simulink model "controllo_test"  (R2020a)
settings: Solver=VariableStepAuto  StartTime=0.0  StopTime=100  RelTol=1e-3
values from neighbouring files (symbols this model uses):
  a = 0.35    [data.m]    (also in geodetic2nedS.m = 6378137)
  a1 = rho * D^4 * alpha1    (= 0.000388302366464)    [data.m]
  a2 = -rho * D^3 * alpha2 * (1 - omega)    (= 0.0037030698432)    [data.m]
  AHRS_bias = [0 0 0]    [data.m]
  AHRS_sample_time = 1/50    (= 0.02)    [data.m]
  AHRS_var = ([1 1 2] * pi/180).^2    [data.m]
  alpha1 = 0.0113    [data.m]
  alpha2 = -0.0091    [data.m]
  c = son2(1)    [Sonar_id.m]    (also in data.m = 0.19)
  current = [seaCurrent; 0; 0; 0]    [data.m]
  D = 0.076    [data.m]
  dead_zone_limit = 31.5    [data.m]
  DVL_sample_t = 1/12    (= 0.0833333333333)    [data.m]
  DVL_var1 = 0.005^2    (= 2.5e-05)    [data.m]
  DVL_var2 = 0.015^2    (= 0.000225)    [data.m]
  DVL_var3 = 0.023^2    (= 0.000529)    [data.m]
  gps_sample_t = 1    [data.m]
  H = eye(3)    [data.m]    (also in navigation_data.m)
  IMU_sample_time = 1/100    (= 0.01)    [data.m]
  initial = []    [data.m]
  INSP = unicode2native(inspectionDirection)    [data.m]
  Ki_bodypos1 = 0    [parametri_PID.m]
  Ki_bodypos2 = 0    [parametri_PID.m]
  Ki_bodypos3 = 0    [parametri_PID.m]
  Ki_bodypos4 = 0    [parametri_PID.m]
  Ki_bodypos5 = 0    [parametri_PID.m]
  Ki_depth1 = 0    [parametri_PID.m]
  Ki_depth2 = 0    [parametri_PID.m]
  Ki_depth3 = 0    [parametri_PID.m]
  Ki_depth4 = 0    [parametri_PID.m]
  Ki_depth5 = 0    [parametri_PID.m]
  Ki_latvel1 = 0    [parametri_PID.m]
  Ki_latvel2 = 0    [parametri_PID.m]
  Ki_latvel3 = 0    [parametri_PID.m]
  Ki_latvel4 = 0    [parametri_PID.m]
  Ki_latvel5 = 0    [parametri_PID.m]
  Ki_P1 = 0    [parametri_PID.m]
  Ki_P2 = 0    [parametri_PID.m]
  Ki_P3 = 0    [parametri_PID.m]
  Ki_P4 = 0    [parametri_PID.m]
  Ki_P5 = 0    [parametri_PID.m]
  Ki_R1 = 0    [parametri_PID.m]
  Ki_R2 = 0    [parametri_PID.m]
  Ki_R3 = 0    [parametri_PID.m]
  Ki_R4 = 0    [parametri_PID.m]
  Ki_R5 = 0    [parametri_PID.m]
  Ki_rel_or1 = 0    [parametri_PID.m]
  Ki_rel_or2 = 0    [parametri_PID.m]
  Ki_rel_or3 = 0    [parametri_PID.m]
  Ki_rel_or4 = 0    [parametri_PID.m]
  Ki_rel_or5 = 0    [parametri_PID.m]
  Ki_reldist1 = 0    [parametri_PID.m]
  Ki_reldist2 = 0    [parametri_PID.m]
  Ki_reldist3 = 0    [parametri_PID.m]
  Ki_reldist4 = 0    [parametri_PID.m]
  Ki_reldist5 = 0    [parametri_PID.m]
  Ki_surge1 = 0    [parametri_PID.m]
  Ki_surge2 = 0    [parametri_PID.m]
  Ki_surge3 = 0    [parametri_PID.m]
  Ki_surge4 = 0    [parametri_PID.m]
  Ki_surge5 = 0    [parametri_PID.m]
  Ki_yaw1 = 0    [parametri_PID.m]
  Ki_yaw2 = 0    [parametri_PID.m]
  Ki_yaw3 = 0    [parametri_PID.m]
  Ki_yaw4 = 0    [parametri_PID.m]
  Ki_yaw5 = 0    [parametri_PID.m]
  Kp_bodypos1 = 0    [parametri_PID.m]
  Kp_bodypos2 = 2    [parametri_PID.m]
  Kp_bodypos3 = 2    [parametri_PID.m]
  Kp_bodypos4 = 2    [parametri_PID.m]
  Kp_bodypos5 = 2    [parametri_PID.m]
  Kp_depth1 = 0    [parametri_PID.m]
  Kp_depth2 = 2    [parametri_PID.m]
  Kp_depth3 = 2    [parametri_PID.m]
  Kp_depth4 = 2    [parametri_PID.m]
  Kp_depth5 = 2    [parametri_PID.m]
  Kp_latvel1 = 0    [parametri_PID.m]
  Kp_latvel2 = 2    [parametri_PID.m]
  Kp_latvel3 = 2    [parametri_PID.m]
  Kp_latvel4 = 2    [parametri_PID.m]
  Kp_latvel5 = 2    [parametri_PID.m]
  Kp_P1 = 0    [parametri_PID.m]
  Kp_P2 = 2    [parametri_PID.m]
  Kp_P3 = 2    [parametri_PID.m]
  Kp_P4 = 2    [parametri_PID.m]
  Kp_P5 = 2    [parametri_PID.m]
  Kp_R1 = 0    [parametri_PID.m]
  Kp_R2 = 2    [parametri_PID.m]
  Kp_R3 = 2    [parametri_PID.m]
  Kp_R4 = 2    [parametri_PID.m]
  Kp_R5 = 2    [parametri_PID.m]
  Kp_rel_or1 = 0    [parametri_PID.m]
  Kp_rel_or2 = 2    [parametri_PID.m]
  Kp_rel_or3 = 2    [parametri_PID.m]
  Kp_rel_or4 = 2    [parametri_PID.m]
  Kp_rel_or5 = 2    [parametri_PID.m]
  Kp_reldist1 = 0    [parametri_PID.m]
  Kp_reldist2 = 2    [parametri_PID.m]
  Kp_reldist3 = 2    [parametri_PID.m]
  Kp_reldist4 = 2    [parametri_PID.m]
  Kp_reldist5 = 2    [parametri_PID.m]
  Kp_surge1 = 0    [parametri_PID.m]
  Kp_surge2 = 2    [parametri_PID.m]
  Kp_surge3 = 2    [parametri_PID.m]
  Kp_surge4 = 2    [parametri_PID.m]
  Kp_surge5 = 2    [parametri_PID.m]
  Kp_yaw1 = 0.6*6    (= 3.6)    [parametri_PID.m]
  Kp_yaw2 = 2    [parametri_PID.m]
  Kp_yaw3 = 2    [parametri_PID.m]
  Kp_yaw4 = 2    [parametri_PID.m]
  Kp_yaw5 = 2    [parametri_PID.m]
  M = M_rb + M_a    [Masse.m]
  M_inv = inv(M)    [Masse.m]
  n_max = 340    [data.m]
  num_cycle = 5    [data.m]    (also in navigation_data.m)
  omega = 0.1    [data.m]
  ps_sample_t = 0.02    [data.m]
  ps_var = (5000/3)^2    (= 2777777.77778)    [data.m]
  pylonCenter = [ 43.723046 ... (first row only)    [missionB.m]
  pylonRadius = 10    [missionB.m]
  ... (+3 more)
undefined symbols (not defined in the file or in its folder): arrival_point, DiscIntNeverNeededParam, Kd_bodypos2, Kd_bodyposy2, Kd_dist_mis2, Kd_surge2, Kd_yaw1, Ki_bodyposy2, Ki_dist_mis2, Kp_dist_mis2, s_data
libraries: simulink x8
(part 3 of 4)

== system controllo_test/Controller/ROTAZIONE IN SUPERFICIE/PID_YAW ==
  yaw_err : Inport
  "EN8 " : Inport  Port=2
  rel_or_err : Inport  Port=3
  EN7 : Inport  Port=4
  Constant : Constant  Value=0
  Constant1 : Constant  Value=0
  Discrete-Time Integrator : DiscreteIntegrator  ExternalReset=falling  SampleTime=0.1  ICPrevOutput=DiscIntNeverNeededParam  ICPrevScaledInput=DiscIntNeverNeededParam
  Discrete-Time Integrator1 : DiscreteIntegrator  ExternalReset=falling  SampleTime=0.1  ICPrevOutput=DiscIntNeverNeededParam  ICPrevScaledInput=DiscIntNeverNeededParam
  Gain : Gain  Gain=Kp_yaw3
  Gain1 : Gain  Gain=Kp_rel_or3
  Gain2 : Gain  Gain=Ki_yaw3
  Gain3 : Gain  Gain=Ki_rel_or3
  Sum : Sum  Inputs=++|
  Sum1 : Sum  Inputs=++|
  Switch : Switch  Criteria=u2 > Threshold  Threshold=0.5
  Switch1 : Switch  Criteria=u2 > Threshold  Threshold=0.5
  tau_yaw : Outport
  tau_rel_or : Outport  Port=2
  wires:
  Sum/1 -> tau_yaw/1
  Discrete-Time Integrator/1 -> Sum/2
  Switch/1 -> Gain/1, Gain2/1
  yaw_err/1 -> Switch/1
  Gain/1 -> Sum/1
  "EN8 "/1 -> [EN8], Switch/2
  Constant/1 -> Switch/3
  Gain2/1 -> Discrete-Time Integrator/1
  [EN8] -> Discrete-Time Integrator/2
  Discrete-Time Integrator1/1 -> Sum1/2
  [EN7] -> Discrete-Time Integrator1/2
  rel_or_err/1 -> Switch1/1
  EN7/1 -> [EN7], Switch1/2
  Switch1/1 -> Gain1/1, Gain3/1
  Sum1/1 -> tau_rel_or/1
  Constant1/1 -> Switch1/3
  Gain3/1 -> Discrete-Time Integrator1/1
  Gain1/1 -> Sum1/1

== system controllo_test/Env. & Sensor Model/AHRS SENSOR/Accelerometer ==
  note: Noise Density: < 0.14 mg/√Hz
  In1 : Inport
  Band-Limited White Noise : simulink/Sources/Band-Limited White Noise  Cov=acc_noise  Ts=IMU_sample_time  seed=[23341]
  Bias : Bias  Bias=0.0
  Sum : Sum  Inputs=|++
  lin_acc : Outport
  wires:
  Band-Limited White Noise/1 -> Sum/2
  Sum/1 -> lin_acc/1
  Bias/1 -> Sum/1
  In1/1 -> Bias/1

== system controllo_test/Env. & Sensor Model/AHRS SENSOR/Gyroscope ==
  note: Noise Density: 0.0035 °/s √Hz
  In1 : Inport
  Band-Limited White Noise : simulink/Sources/Band-Limited White Noise  Cov=gyro_noise  Ts=IMU_sample_time  seed=[341]
  Bias : Bias  Bias=0.0
  Sum : Sum  Inputs=|++
  ang_vel : Outport
  wires:
  Band-Limited White Noise/1 -> Sum/2
  Sum/1 -> ang_vel/1
  Bias/1 -> Sum/1
  In1/1 -> Bias/1

== system controllo_test/Env. & Sensor Model/AHRS SENSOR/Magnetometer ==
  note: Noise Density: 140 μGauss/√Hz
  In1 : Inport
  Band-Limited White Noise : simulink/Sources/Band-Limited White Noise  Cov=magn_noise  Ts=IMU_sample_time  seed=[31]
  Bias : Bias  Bias=0.0
  Sum : Sum  Inputs=|++
  m : Outport
  wires:
  Band-Limited White Noise/1 -> Sum/2
  Sum/1 -> m/1
  Bias/1 -> Sum/1
  In1/1 -> Bias/1

== system controllo_test/Env. & Sensor Model/DVL SENSOR/Subsystem ==
  In1 : Inport
  Abs : Abs
  Random Number : RandomNumber  Variance=DVL_var3  Seed=1  SampleTime=DVL_sample_t
  Random Number1 : RandomNumber  Variance=DVL_var2  Seed=2  SampleTime=DVL_sample_t
  Random Number2 : RandomNumber  Variance=DVL_var1  Seed=3  SampleTime=DVL_sample_t
  Switch2 : Switch  Criteria=u2 > Threshold  Threshold=2
  Switch3 : Switch  Criteria=u2 > Threshold  Threshold=4
  Out1 : Outport
  wires:
  Switch3/1 -> Switch2/1
  Random Number1/1 -> Switch3/3
  Random Number2/1 -> Switch2/3
  In1/1 -> Abs/1
  Switch2/1 -> Out1/1
  Random Number/1 -> Switch3/1
  Abs/1 -> Switch3/2, Switch2/2

== system controllo_test/Env. & Sensor Model/DVL SENSOR/Subsystem1 ==
  In1 : Inport
  Abs : Abs
  Random Number : RandomNumber  Variance=DVL_var3  Seed=4  SampleTime=DVL_sample_t
  Random Number1 : RandomNumber  Variance=DVL_var2  Seed=5  SampleTime=DVL_sample_t
  Random Number2 : RandomNumber  Variance=DVL_var1  Seed=2  SampleTime=DVL_sample_t
  Switch2 : Switch  Criteria=u2 > Threshold  Threshold=2
  Switch3 : Switch  Criteria=u2 > Threshold  Threshold=4
  Out1 : Outport
  wires:
  Switch3/1 -> Switch2/1
  Random Number1/1 -> Switch3/3
  Random Number2/1 -> Switch2/3
  In1/1 -> Abs/1
  Switch2/1 -> Out1/1
  Random Number/1 -> Switch3/1
  Abs/1 -> Switch3/2, Switch2/2

== system controllo_test/Env. & Sensor Model/DVL SENSOR/Subsystem2 ==
  In1 : Inport
  Abs : Abs
  Random Number : RandomNumber  Variance=DVL_var3  Seed=7  SampleTime=DVL_sample_t
  Random Number1 : RandomNumber  Variance=DVL_var2  Seed=2  SampleTime=DVL_sample_t
  Random Number2 : RandomNumber  Variance=DVL_var1  Seed=1  SampleTime=DVL_sample_t
  Switch2 : Switch  Criteria=u2 > Threshold  Threshold=2
  Switch3 : Switch  Criteria=u2 > Threshold  Threshold=4
  Out1 : Outport
  wires:
  Switch3/1 -> Switch2/1
  Random Number1/1 -> Switch3/3
  Random Number2/1 -> Switch2/3
  In1/1 -> Abs/1
  Switch2/1 -> Out1/1
  Random Number/1 -> Switch3/1
  Abs/1 -> Switch3/2, Switch2/2

== system controllo_test/Env. & Sensor Model/GPS SENSOR/Add noiose ==
  In1 : Inport
  In2 : Inport  Port=2
  Bus Creator : BusCreator  Inputs=2
  Random Number : RandomNumber  Variance=2  SampleTime=1
  Random Number1 : RandomNumber  Variance=2  Seed=332  SampleTime=1
  Sum2 : Sum  Inputs=|++
  Sum3 : Sum  Inputs=|++
  Out1 : Outport
  wires:
  In2/1 -> Sum3/1  "y in"
  Bus Creator/1 -> Out1/1  "out"
  In1/1 -> Sum2/1  "x in"
  Random Number/1 -> Sum2/2  "noise x"
  Random Number1/1 -> Sum3/2  "noise y"
  Sum2/1 -> Bus Creator/1  "x out"
  Sum3/1 -> Bus Creator/2  "y out"

== system controllo_test/Env. & Sensor Model/GPS SENSOR/Control state ==
  In1 : Inport
  AND : Logic  IconShape=distinctive  AllPortsSameDT=off  OutDataTypeStr=boolean
  Data Type Conversion : DataTypeConversion  OutDataTypeStr=double
  ENABLE GPS : Constant
  Zero-Order Hold : ZeroOrderHold  SampleTime=gps_sample_t
  Flag enable gps : Outport
  wires:
  ENABLE GPS/1 -> AND/2
  In1/1 -> AND/1
  AND/1 -> Data Type Conversion/1
  Data Type Conversion/1 -> Zero-Order Hold/1
  Zero-Order Hold/1 -> Flag enable gps/1

== system controllo_test/Env. & Sensor Model/Sonar sensor/Noises ==
  Mux : Mux  Inputs=s_data.num
  Random Number : RandomNumber  Mean=s_data.bias  Variance=s_data.noise^2  Seed=1  SampleTime=s_data.smpl  VectorParams1D=off
  Random Number1 : RandomNumber  Mean=s_data.bias  Variance=s_data.noise^2  Seed=2  SampleTime=s_data.smpl  VectorParams1D=off
  Random Number2 : RandomNumber  Mean=s_data.bias  Variance=s_data.noise^2  Seed=3  SampleTime=s_data.smpl  VectorParams1D=off
  Random Number3 : RandomNumber  Mean=s_data.bias  Variance=s_data.noise^2  Seed=4  SampleTime=s_data.smpl  VectorParams1D=off
  Random Number4 : RandomNumber  Mean=s_data.bias  Variance=s_data.noise^2  Seed=5  SampleTime=s_data.smpl  VectorParams1D=off
  Noises : Outport  SampleTime=s_data.smpl
  wires:
  Mux/1 -> Noises/1
  Random Number/1 -> Mux/1
  Random Number1/1 -> Mux/2
  Random Number2/1 -> Mux/3
  Random Number3/1 -> Mux/4
  Random Number4/1 -> Mux/5

== system controllo_test/Navigation1/Relative estimation/Sonar trigger ==
  In1 : Inport
  Demux : Demux  Outputs=[5 5]
  MATLAB Function : MATLAB Function  TreatAsAtomicUnit=on
  Scope2 : Scope
  Sum : Sum  Inputs=|+-
  Terminator : Terminator
  prev_sonar : Memory  InitialCondition=zeros(5,1)
  Out2 : Outport
  wires:
  Sum/1 -> MATLAB Function/2(sum)
  prev_sonar/1 -> Sum/2
  MATLAB Function/1(pulse) -> Out2/1, Scope2/1
  Demux/2 -> Terminator/1
  MATLAB Function/2(prev) -> prev_sonar/1
  In1/1 -> Demux/1
  Demux/1 -> MATLAB Function/1(sonar), Sum/1

== system controllo_test/Navigation1/Relative estimation/Subsystem ==
  Sonar : Inport
  Orientation : Inport  Port=2
  Trigger : TriggerPort  VariantControl=Variant  PortDimensions=1
  Demux : Demux  Outputs=[5 5]
  Display : Display
  Display1 : Display
  MATLAB Function9 : MATLAB Function  TreatAsAtomicUnit=on
  Terminator : Terminator
  Rel_distance : Outport  PortDimensions=1
  Rel_angle : Outport  Port=2  PortDimensions=1
  flag_sonar : Outport  Port=3  PortDimensions=1
  wires:
  Sonar/1 -> Demux/1, MATLAB Function9/1(sonar)
  MATLAB Function9/3(flag_sonar) -> Display/1, flag_sonar/1
  Orientation/1 -> MATLAB Function9/2(orientation)
  MATLAB Function9/2(alpha) -> Rel_angle/1
  MATLAB Function9/1(distance) -> Rel_distance/1
  Demux/1 -> Terminator/1
  Demux/2 -> Display1/1

== system controllo_test/Navigation1/z_EKF/EXTENDED KALMAN FILTER ==
  dT : Inport
  init : Inport  Port=2
  P0 : Inport  Port=3
  meas_pos : Inport  Port=4
  GPS_flag : Inport  Port=5
  meas_depth : Inport  Port=6
  orientation : Inport  Port=7
  dvl : Inport  Port=8
  ahrs_flag : Inport  Port=9
  Trigger : TriggerPort  VariantControl=Variant  PortDimensions=1
  "Correzione " : MATLAB Function  TreatAsAtomicUnit=on
  Demux : Demux  Outputs=[2 1]
  P : Memory  InitialCondition=zeros(3)  InheritSampleTime=on  StateName=P_pos
  Predizione : MATLAB Function  TreatAsAtomicUnit=on
  Scope : Scope
  hat_ : Memory  InitialCondition=zeros(3,1)  InheritSampleTime=on  StateName=P_pos
  previous_pos : Memory  InitialCondition=zeros(2,1)  InheritSampleTime=on  StateName=P_pos
  hat_pos : Outport
  hat_depth : Outport  Port=2
  wires:
  P/1 -> Predizione/1("P ")
  "Correzione "/2(P) -> P/1, Scope/1
  "Correzione "/1(prev_pos) -> previous_pos/1
  hat_/1 -> Predizione/2("hat ")
  "Correzione "/3(hat) -> Demux/1, hat_/1
  previous_pos/1 -> "Correzione "/1("prev_pos ")
  init/1 -> Predizione/7(init)
  orientation/1 -> Predizione/4(orientation)
  dT/1 -> Predizione/3(dT)
  dvl/1 -> Predizione/5(dvl)
  ahrs_flag/1 -> Predizione/6(ahrs_flag)
  P0/1 -> Predizione/8(P0)
  Predizione/1(P) -> "Correzione "/2("P ")
  Predizione/2(hat) -> "Correzione "/3("hat ")
  meas_pos/1 -> "Correzione "/4(meas_pos)
  GPS_flag/1 -> "Correzione "/5(GPS_flag)
  Demux/1 -> hat_pos/1
  Demux/2 -> hat_depth/1
  meas_depth/1 -> "Correzione "/6(meas_depth)

== system controllo_test/Navigation1/z_EKF/Trigger & Init ==
  meas_depth : Inport
  "meas_pos " : Inport  Port=2
  AND : Logic  IconShape=distinctive  AllPortsSameDT=off  OutDataTypeStr=boolean
  Depth trigger : Subsystem
  Initialization : Subsystem
  Scope{,1..3} (4 alike) : Scope
  pulse : Outport
  dT : Outport  Port=2
  init : Outport  Port=3
  P0 : Outport  Port=4
  wires:
  meas_depth/1 -> Depth trigger/1(Meas_depth), Initialization/1(Meas_depth)
  Depth trigger/2(Pulse) -> AND/1, Scope2/1
  "meas_pos "/1 -> Initialization/2(Meas_pos)
  Initialization/2(init) -> init/1, Scope3/1
  Initialization/3(P0) -> Scope/1, P0/1
  Depth trigger/1(dT) -> dT/1
  Initialization/1(pulse) -> AND/2, Scope1/1
  AND/1 -> pulse/1

== system controllo_test/Vehicle Model/Model Vehicle/Kinematic ==
  eta : Inport
  ni : Inport  Port=2
  Jac : MATLAB Function  TreatAsAtomicUnit=on
  Product : Product  Multiplication=Matrix(*)
  eta_dot : Outport  VectorParamsAs1DForOutWhenUnconnected=off
  wires:
  ni/1 -> Product/2
  Jac/1(J) -> Product/1
  eta/1 -> Jac/1(eta)
  Product/1 -> eta_dot/1

== system controllo_test/Vehicle Model/Thrusters/T ==
  des rot : Inport
  ni : Inport  Port=2
  Demux : Demux  Outputs=7
  Demux1 : Demux  Outputs=7
  MATLAB Function : MATLAB Function  TreatAsAtomicUnit=on
  Mux : Mux  Inputs=7
  Thruster 1 : Subsystem
  Thruster 2 : Subsystem
  Thruster 3 : Subsystem
  Thruster 4 : Subsystem
  Thruster 5 : Subsystem
  Thruster 6 : Subsystem
  Thruster 7 : Subsystem
  T : Outport  VectorParamsAs1DForOutWhenUnconnected=off
  wires:
  Demux/1 -> Thruster 1/1(n [rad/s])
  Demux/2 -> Thruster 2/1(n [rad/s])
  Demux/3 -> Thruster 3/1(n [rad/s])
  Demux/4 -> Thruster 4/1(n [rad/s])
  Demux/5 -> Thruster 5/1(n [rad/s])
  Demux/6 -> Thruster 6/1(n [rad/s])
  Demux/7 -> Thruster 7/1(n [rad/s])
  des rot/1 -> Demux/1
  Thruster 7/1(T i) -> Mux/7
  Thruster 6/1(T i) -> Mux/6
  Thruster 5/1(T i) -> Mux/5
  Thruster 4/1(T i) -> Mux/4
  Thruster 3/1(T i) -> Mux/3
  Thruster 2/1(T i) -> Mux/2
  Thruster 1/1(T i) -> Mux/1
  Mux/1 -> T/1
  MATLAB Function/1(v_th) -> Demux1/1
  Demux1/1 -> Thruster 1/2(V [m/s])
  Demux1/2 -> Thruster 2/2(V [m/s])
  Demux1/3 -> Thruster 3/2(V [m/s])
  Demux1/4 -> Thruster 4/2(V [m/s])
  Demux1/5 -> Thruster 5/2(V [m/s])
  Demux1/6 -> Thruster 6/2(V [m/s])
  Demux1/7 -> Thruster 7/2(V [m/s])
  ni/1 -> MATLAB Function/1(ni)

== system controllo_test/Navigation1/z_EKF/Trigger & Init/Depth trigger ==
  Meas_depth : Inport
  Demux : Demux  Outputs=2
  MATLAB Function : MATLAB Function  TreatAsAtomicUnit=on
  Sum : Sum  Inputs=|+-
  Terminator : Terminator
  count : Memory  InitialCondition=1
  prev_depth : Memory
  dT : Outport
  Pulse : Outport  Port=2
  wires:
  Sum/1 -> MATLAB Function/3(sum)
  prev_depth/1 -> Sum/2
  MATLAB Function/3(pulse) -> Pulse/1
  Demux/2 -> Terminator/1
  MATLAB Function/4(prev) -> prev_depth/1
  MATLAB Function/2(dT) -> dT/1
  Meas_depth/1 -> Demux/1
  count/1 -> MATLAB Function/1("count ")
  Demux/1 -> MATLAB Function/2(depth), Sum/1
  MATLAB Function/1(count) -> count/1

== system controllo_test/Navigation1/z_EKF/Trigger & Init/Initialization ==
  Meas_depth : Inport
  Meas_pos : Inport  Port=2
  Demux1 : Demux  Outputs=[2 1]
  Demux2 : Demux  Outputs=2
  MATLAB Function1 : MATLAB Function  TreatAsAtomicUnit=on
  Scope3 : Scope
  Sum1 : Sum  Inputs=|+-
  Terminator2 : Terminator
  init_counter : Memory
  prev_pos : Memory  InitialCondition=zeros(2,1)
  store_depth : Memory  InitialCondition=zeros(num_cycle,1)
  store_gps : Memory  InitialCondition=zeros(2,num_cycle)
  pulse : Outport
  init : Outport  Port=2
  P0 : Outport  Port=3
  wires:
  Demux1/1 -> MATLAB Function1/3(gps), Sum1/1
  MATLAB Function1/4(P0) -> P0/1
  MATLAB Function1/3(init) -> init/1
  MATLAB Function1/2(pulse) -> pulse/1, Scope3/1
  init_counter/1 -> MATLAB Function1/1("init_counter ")
  Sum1/1 -> MATLAB Function1/5(diff_)
  Demux2/1 -> MATLAB Function1/2(depth)
  MATLAB Function1/6(gps_store) -> store_gps/1
  MATLAB Function1/1(init_counter) -> init_counter/1
  Demux2/2 -> Terminator2/1
  MATLAB Function1/7(depth_store) -> store_depth/1
  store_gps/1 -> MATLAB Function1/6(store_gps)
  store_depth/1 -> MATLAB Function1/7(store_depth)
  Meas_depth/1 -> Demux2/1
  MATLAB Function1/5(prev) -> prev_pos/1
  prev_pos/1 -> Sum1/2
  Meas_pos/1 -> Demux1/1
  Demux1/2 -> MATLAB Function1/4(GPS_flag)

== system controllo_test/Vehicle Model/Thrusters/T/Thruster 1 ==
  note: n is the rotational speed of the thruster
      | V is the speed component of the water along the thruster axis
      |
      | n is saturated according to data
      | a dead zone is considered according to data
      | the thruster is characterised by 1st order dynamics (tau = 0.2s)
  n [rad/s] : Inport
  V [m/s] : Inport  Port=2
  Dead Zone : DeadZone  LowerValue=-dead_zone_limit  UpperValue=dead_zone_limit  SaturateOnIntegerOverflow=on
  MATLAB Function : MATLAB Function  TreatAsAtomicUnit=on
  Saturation : Saturate  UpperLimit=n_max  LowerLimit=-n_max
  Transfer Fcn : TransferFcn  Denominator=[0.2 1]
  T i : Outport
  wires:
  V [m/s]/1 -> MATLAB Function/2(V)
  Saturation/1 -> MATLAB Function/1(n)
  Transfer Fcn/1 -> Saturation/1
  Dead Zone/1 -> Transfer Fcn/1
  n [rad/s]/1 -> Dead Zone/1
  MATLAB Function/1(T) -> T i/1

== system controllo_test/Vehicle Model/Thrusters/T/Thruster 2 ==
  note: n is the rotational speed of the thruster
      | V is the speed component of the water along the thruster axis
      |
      | n is saturated according to data
      | a dead zone is considered according to data
      | the thruster is characterised by 1st order dynamics (tau = 0.2s)
  n [rad/s] : Inport
  V [m/s] : Inport  Port=2
  Dead Zone : DeadZone  LowerValue=-dead_zone_limit  UpperValue=dead_zone_limit  SaturateOnIntegerOverflow=on
  MATLAB Function : MATLAB Function  TreatAsAtomicUnit=on
  Saturation : Saturate  UpperLimit=n_max  LowerLimit=-n_max
  Transfer Fcn : TransferFcn  Denominator=[0.2 1]
  T i : Outport
  wires:
  V [m/s]/1 -> MATLAB Function/2(V)
  Saturation/1 -> MATLAB Function/1(n)
  Transfer Fcn/1 -> Saturation/1
  Dead Zone/1 -> Transfer Fcn/1
  n [rad/s]/1 -> Dead Zone/1
  MATLAB Function/1(T) -> T i/1

== system controllo_test/Vehicle Model/Thrusters/T/Thruster 3 ==
  note: n is the rotational speed of the thruster
      | V is the speed component of the water along the thruster axis
      |
      | n is saturated according to data
      | a dead zone is considered according to data
      | the thruster is characterised by 1st order dynamics (tau = 0.2s)
  n [rad/s] : Inport
  V [m/s] : Inport  Port=2
  Dead Zone : DeadZone  LowerValue=-dead_zone_limit  UpperValue=dead_zone_limit  SaturateOnIntegerOverflow=on
  MATLAB Function : MATLAB Function  TreatAsAtomicUnit=on
  Saturation : Saturate  UpperLimit=n_max  LowerLimit=-n_max
  Transfer Fcn : TransferFcn  Denominator=[0.2 1]
  T i : Outport
  wires:
  V [m/s]/1 -> MATLAB Function/2(V)
  Saturation/1 -> MATLAB Function/1(n)
  Transfer Fcn/1 -> Saturation/1
  Dead Zone/1 -> Transfer Fcn/1
  n [rad/s]/1 -> Dead Zone/1
  MATLAB Function/1(T) -> T i/1

== system controllo_test/Vehicle Model/Thrusters/T/Thruster 4 ==
  note: n is the rotational speed of the thruster
      | V is the speed component of the water along the thruster axis
      |
      | n is saturated according to data
      | a dead zone is considered according to data
      | the thruster is characterised by 1st order dynamics (tau = 0.2s)
  n [rad/s] : Inport
  V [m/s] : Inport  Port=2
  Dead Zone : DeadZone  LowerValue=-dead_zone_limit  UpperValue=dead_zone_limit  SaturateOnIntegerOverflow=on
  MATLAB Function : MATLAB Function  TreatAsAtomicUnit=on
  Saturation : Saturate  UpperLimit=n_max  LowerLimit=-n_max
  Transfer Fcn : TransferFcn  Denominator=[0.2 1]
  T i : Outport
  wires:
  V [m/s]/1 -> MATLAB Function/2(V)
  Saturation/1 -> MATLAB Function/1(n)
  Transfer Fcn/1 -> Saturation/1
  Dead Zone/1 -> Transfer Fcn/1
  n [rad/s]/1 -> Dead Zone/1
  MATLAB Function/1(T) -> T i/1

== system controllo_test/Vehicle Model/Thrusters/T/Thruster 5 ==
  note: n is the rotational speed of the thruster
      | V is the speed component of the water along the thruster axis
      |
      | n is saturated according to data
      | a dead zone is considered according to data
      | the thruster is characterised by 1st order dynamics (tau = 0.2s)
  n [rad/s] : Inport
  V [m/s] : Inport  Port=2
  Dead Zone : DeadZone  LowerValue=-dead_zone_limit  UpperValue=dead_zone_limit  SaturateOnIntegerOverflow=on
  MATLAB Function : MATLAB Function  TreatAsAtomicUnit=on
  Saturation : Saturate  UpperLimit=n_max  LowerLimit=-n_max
  Transfer Fcn : TransferFcn  Denominator=[0.2 1]
  T i : Outport
  wires:
  V [m/s]/1 -> MATLAB Function/2(V)
  Saturation/1 -> MATLAB Function/1(n)
  Transfer Fcn/1 -> Saturation/1
  Dead Zone/1 -> Transfer Fcn/1
  n [rad/s]/1 -> Dead Zone/1
  MATLAB Function/1(T) -> T i/1

== system controllo_test/Vehicle Model/Thrusters/T/Thruster 6 ==
  note: n is the rotational speed of the thruster
      | V is the speed component of the water along the thruster axis
      |
      | n is saturated according to data
      | a dead zone is considered according to data
      | the thruster is characterised by 1st order dynamics (tau = 0.2s)
  n [rad/s] : Inport
  V [m/s] : Inport  Port=2
  Dead Zone : DeadZone  LowerValue=-dead_zone_limit  UpperValue=dead_zone_limit  SaturateOnIntegerOverflow=on
  MATLAB Function : MATLAB Function  TreatAsAtomicUnit=on
  Saturation : Saturate  UpperLimit=n_max  LowerLimit=-n_max
  Transfer Fcn : TransferFcn  Denominator=[0.2 1]
  T i : Outport
  wires:
  V [m/s]/1 -> MATLAB Function/2(V)
  Saturation/1 -> MATLAB Function/1(n)
  Transfer Fcn/1 -> Saturation/1
  Dead Zone/1 -> Transfer Fcn/1
  n [rad/s]/1 -> Dead Zone/1
  MATLAB Function/1(T) -> T i/1

== system controllo_test/Vehicle Model/Thrusters/T/Thruster 7 ==
  note: n is the rotational speed of the thruster
      | V is the speed component of the water along the thruster axis
      |
      | n is saturated according to data
      | a dead zone is considered according to data
      | the thruster is characterised by 1st order dynamics (tau = 0.2s)
  n [rad/s] : Inport
  V [m/s] : Inport  Port=2
  Dead Zone : DeadZone  LowerValue=-dead_zone_limit  UpperValue=dead_zone_limit  SaturateOnIntegerOverflow=on
  MATLAB Function : MATLAB Function  TreatAsAtomicUnit=on
  Saturation : Saturate  UpperLimit=n_max  LowerLimit=-n_max
  Transfer Fcn : TransferFcn  Denominator=[0.2 1]
  T i : Outport
  wires:
  V [m/s]/1 -> MATLAB Function/2(V)
  Saturation/1 -> MATLAB Function/1(n)
  Transfer Fcn/1 -> Saturation/1
  Dead Zone/1 -> Transfer Fcn/1
  n [rad/s]/1 -> Dead Zone/1
  MATLAB Function/1(T) -> T i/1

== matlab function controllo_test/Vehicle Model/Thrusters/T/Thruster 3/MATLAB Function ==
  data: n input; T output; V input; D parameter; omega parameter; a1 parameter; a2 parameter; alpha1 parameter; alpha2 parameter
function T = thrusterModel(n, V, D, omega, a1, a2, alpha1, alpha2)

Va = (1-omega) * V;     % Advancement velocity at the propeller
J0 = Va/(n*D);          % Advancement Coefficient

if J0 > -alpha1/alpha2  % Out of linearity domain (right side)
    T = 0;              % A null generated thrust is assumed
    
elseif J0 < 0           % Out of linearity domain (left side)
    T = a1*abs(n)*n;    % Bollard thrust is assumed

else                    % Within the linearity domain
    T = a1*abs(n)*n - a2*abs(n)*V;
end

== matlab function controllo_test/Vehicle Model/Thrusters/T/Thruster 4/MATLAB Function ==
  data: n input; T output; V input; D parameter; omega parameter; a1 parameter; a2 parameter; alpha1 parameter; alpha2 parameter
function T = thrusterModel(n, V, D, omega, a1, a2, alpha1, alpha2)

Va = (1-omega) * V;     % Advancement velocity at the propeller
J0 = Va/(n*D);          % Advancement Coefficient

if J0 > -alpha1/alpha2  % Out of linearity domain (right side)
    T = 0;              % A null generated thrust is assumed
    
elseif J0 < 0           % Out of linearity domain (left side)
    T = a1*abs(n)*n;    % Bollard thrust is assumed

else                    % Within the linearity domain
    T = a1*abs(n)*n - a2*abs(n)*V;
end

== matlab function controllo_test/Vehicle Model/Thrusters/T/Thruster 5/MATLAB Function ==
  data: n input; T output; V input; D parameter; omega parameter; a1 parameter; a2 parameter; alpha1 parameter; alpha2 parameter
function T = thrusterModel(n, V, D, omega, a1, a2, alpha1, alpha2)

Va = (1-omega) * V;     % Advancement velocity at the propeller
J0 = Va/(n*D);          % Advancement Coefficient

if J0 > -alpha1/alpha2  % Out of linearity domain (right side)
    T = 0;              % A null generated thrust is assumed
    
elseif J0 < 0           % Out of linearity domain (left side)
    T = a1*abs(n)*n;    % Bollard thrust is assumed

else                    % Within the linearity domain
    T = a1*abs(n)*n - a2*abs(n)*V;
end

== matlab function controllo_test/Vehicle Model/Thrusters/T/Thruster 6/MATLAB Function ==
  data: n input; T output; V input; D parameter; omega parameter; a1 parameter; a2 parameter; alpha1 parameter; alpha2 parameter
function T = thrusterModel(n, V, D, omega, a1, a2, alpha1, alpha2)

Va = (1-omega) * V;     % Advancement velocity at the propeller
J0 = Va/(n*D);          % Advancement Coefficient

if J0 > -alpha1/alpha2  % Out of linearity domain (right side)
    T = 0;              % A null generated thrust is assumed
    
elseif J0 < 0           % Out of linearity domain (left side)
    T = a1*abs(n)*n;    % Bollard thrust is assumed

else                    % Within the linearity domain
    T = a1*abs(n)*n - a2*abs(n)*V;
end

== matlab function controllo_test/Vehicle Model/Thrusters/T/Thruster 7/MATLAB Function ==
  data: n input; T output; V input; D parameter; omega parameter; a1 parameter; a2 parameter; alpha1 parameter; alpha2 parameter
function T = thrusterModel(n, V, D, omega, a1, a2, alpha1, alpha2)

Va = (1-omega) * V;     % Advancement velocity at the propeller
J0 = Va/(n*D);          % Advancement Coefficient

if J0 > -alpha1/alpha2  % Out of linearity domain (right side)
    T = 0;              % A null generated thrust is assumed
    
elseif J0 < 0           % Out of linearity domain (left side)
    T = a1*abs(n)*n;    % Bollard thrust is assumed

else                    % Within the linearity domain
    T = a1*abs(n)*n - a2*abs(n)*V;
end

== matlab function controllo_test/Vehicle Model/Model Vehicle/MATLAB Function ==
  data: coord_pylon input; eta input; eta_ecef output
function eta_ecef = nedToEcef(coord_pylon, eta)

    coder.extrinsic('wgs84Ellipsoid');

    coder.extrinsic('ned2geodetic');
    
    eta_pos = eta(1:6);
    wgs84 = wgs84Ellipsoid('meter'); %TODO verificare che esprima le coordinate nello stesso modo dell'ECEF dato in missionB.m
    [eta_pos(1), eta_pos(2)] = ned2geodetic(eta(1), eta(2), eta(3), coord_pylon(1), coord_pylon(2), coord_pylon(3), wgs84,'degrees');
    
    eta_pos(3) = eta(3);
    eta_pos(4:6) = eta_pos(4:6);
    
    eta_ecef = eta_pos;
    
end

== matlab function controllo_test/Vehicle Model/MATLAB Function ==
  data: eta input; ni_c output; current input
function ni_c = current_ned2body(eta, current)
    eta2 = eta(4:6)*pi/180;     % eta2 espresso in radianti
    ni_c = Jac(eta2)'*current;
end

== matlab function controllo_test/Vehicle Model/Thrusters/T/MATLAB Function ==
  data: ni input; v_th output
function v_th = thrusters(ni)
p1 = [-0.35 -0.25 0]';
p2 = [-0.35 0.25 0]';
p3 = [-0.25 -0.35 0]';
p4 = [0.25 0.35 0]';
p5 = [-0.25 -0.25 -0.19]';
p6 = [-0.25 0.25 -0.19]';
p7 = [0.25 0 -0.19]';

t1 = [1 0 0]';
t2 = t1;
t3 = [0 1 0]';
t4 = -t3;
t5 = [0 0 1]';
t6 = t5;
t7 = t5;

v_lin = ni(1:3);
v_ang = ni(4:6);

vp1 = v_lin + cross(v_ang, p1);
vp2 = v_lin + cross(v_ang, p2);
vp3 = v_lin + cross(v_ang, p3);
vp4 = v_lin + cross(v_ang, p4);
vp5 = v_lin + cross(v_ang, p5);
vp6 = v_lin + cross(v_ang, p6);
vp7 = v_lin + cross(v_ang, p7);

v1 = vp1'*t1;
v2 = vp2'*t2;
v3 = vp3'*t3;
v4 = vp4'*t4;
v5 = vp5'*t5;
v6 = vp6'*t6;
v7 = vp7'*t7;

v_th = [ v1 v2 v3 v4 v5 v6 v7]';
end

== matlab function controllo_test/Navigation1/Geodetic to NED/MATLAB Function2 ==
  data: GPS_geodetic input; GPS_flag input; GPS_NED output; depth input; pylonCenter parameter
function GPS_NED = Geo2NED(GPS_geodetic, GPS_flag, depth, pylonCenter)

% Funzione che trasforma le coordinate dal sistema di riferimento geodetico
% ad un sistema NED con origine in corrispondenza del centro del pilone.

%% GPS non funzionante
if GPS_flag == 0            
    GPS_NED = [0;0;0];
    return
end

%% Variabili
phi = GPS_geodetic(1);                  % Coordinate geodetiche in radianti                     
lambda = GPS_geodetic(2);  
h = -depth;

phi_pyl = pylonCenter(1) * pi/180;      % Origine del sistema NED in coordinate geodetiche
lambda_pyl = pylonCenter(2) * pi/180;

%% Trasformazione coordinate
coder.extrinsic('wgs84Ellipsoid');
coder.extrinsic('geodetic2ned');
    
[x_gps2, y_gps2, z_gps2] = geodetic2ned(phi, lambda, -depth, phi_pyl, lambda_pyl, 0, wgs84Ellipsoid, 'radians');
eta_NED_GPS = [x_gps2; y_gps2];

GPS_NED = zeros(3,1);
GPS_NED(1) = eta_NED_GPS(1);            % Coordiante NED in radianti
GPS_NED(2) = eta_NED_GPS(2);
GPS_NED(3) = GPS_flag;

== matlab function controllo_test/Vehicle Model/Thrusters/saturation_tau ==
  data: tau input; tau_sat output; eta input
function tau_sat = sat_tau(tau, eta)
    tau_sat = [0;0;0;0;0;0];
    tau_sat = tau;

    if eta(3) < 0.1 %semiasse c
        tau_sat(3) = 0;
    end
    
end

== matlab function controllo_test/Navigation1/Geodetic to NED2/MATLAB Function2 ==
  data: GPS_geodetic input; GPS_flag input; GPS_NED output; depth input; pylonCenter parameter
function GPS_NED = Geo2NED(GPS_geodetic, GPS_flag, depth, pylonCenter)

% Funzione che trasforma le coordinate dal sistema di riferimento geodetico
% ad un sistema NED con origine in corrispondenza del centro del pilone.

%% GPS non funzionante
if GPS_flag == 0            
    GPS_NED = [0;0;0];
    return
end

%% Variabili
phi = GPS_geodetic(1);                  % Coordinate geodetiche in radianti                     
lambda = GPS_geodetic(2);  
h = -depth;

phi_pyl = pylonCenter(1) * pi/180;      % Origine del sistema NED in coordinate geodetiche
lambda_pyl = pylonCenter(2) * pi/180;

%% Trasformazione coordinate
coder.extrinsic('wgs84Ellipsoid');
coder.extrinsic('geodetic2ned');
    
[x_gps2, y_gps2, z_gps2] = geodetic2ned(phi, lambda, -depth, phi_pyl, lambda_pyl, 0, wgs84Ellipsoid, 'radians');
eta_NED_GPS = [x_gps2; y_gps2];

GPS_NED = zeros(3,1);
GPS_NED(1) = eta_NED_GPS(1);            % Coordiante NED in radianti
GPS_NED(2) = eta_NED_GPS(2);
GPS_NED(3) = GPS_flag;

== matlab function controllo_test/Navigation1/MATLAB Function1 ==
  data: ang_vel input; DVL input; nu_1 output; c parameter
function nu_1  = dvl2body(ang_vel, DVL, c)

% Funzione che si occupa di trasformare la velocità da sistema di
% riferimento associato al DVL al sistema BODY

% nu_dvl = R_b^dvl (nu_1 + S(nu_2)* P_dvl)
% nu_1 = R_b^dvl' * nu_dvl - S(nu_2) * P_dvl

nu_1    =   zeros(4,1);
nu_2    =   [ang_vel(1); ang_vel(2); ang_vel(3)];
vel_dvl =   [DVL(1); DVL(2); DVL(3)];
R_b_dvl =   eye(3);

S = [   0,          -nu_2(3),   nu_2(2); 
        nu_2(3),    0,          -nu_2(1); 
        -nu_2(2),   nu_2(1),    0       ];
    
p = [0;0;c];

nu_1(1:3) = R_b_dvl' * vel_dvl - S * p;
nu_1(4) = DVL(4); %Flag

== matlab function controllo_test/Navigation1/MATLAB Function2 ==
  data: Depth_ps input; Depth output; c parameter
function  Depth = ps2body(Depth_ps, c)
% Il profondimetro è posizionato nella parte inferiore dell'AUV, lungo
% l'asse z
Depth = zeros(2,1);
Depth(1) = Depth_ps(1) - c;     %profondità rispetto al centro di massa
Depth(2) = Depth_ps(2);         %flag

== matlab function controllo_test/Navigation1/AHRS_function ==
  data: eta2 output; lin_acc input; nu2 output; ang_vel input; orientation input
function [eta2, nu2]= AHRS_signals(lin_acc, ang_vel, orientation)
acc = lin_acc(1:3);
nu2 = ang_vel(1:3);
eta2 = orientation(1:3);

== matlab function controllo_test/Navigation1/DVL_function ==
  data: dvl input; velocity_est output; flag_DVL output
function [velocity_est, flag_DVL] = DVL_signals(dvl)
velocity_est = dvl(1:3);
flag_DVL = dvl(4);

== matlab function controllo_test/Navigation1/NED to Geodetic/MATLAB Function1 ==
  data: eta_NED input; eta_geodetic output; depth input; pylonCenter parameter
function eta_geodetic = NED2Geo(eta_NED, depth, pylonCenter)

% Funzione che trasforma le coordinate dal sistema NED con origine in
% corrispondenza del centro del pilone al sistema di riferimento geodetico

phi_pyl = pylonCenter(1) * pi/180;      % Origine del sistema NED in coordinate geodetiche 
lambda_pyl = pylonCenter(2) * pi/180;

%% Trasformazione
coder.extrinsic('wgs84Ellipsoid');
coder.extrinsic('ned2geodetic');

[lat, lon, h] = ned2geodetic(eta_NED(1), eta_NED(2), depth, phi_pyl, lambda_pyl, 0, wgs84Ellipsoid, 'radians');

eta_geodetic = [0; 0];
eta_geodetic = [lat; lon];              % Coordiante geodetiche in radianti

== matlab function controllo_test/Navigation1/Relative estimation/Sonar trigger/MATLAB Function ==
  data: sonar input; sum input; pulse output; prev output
function [pulse, prev] = fcn(sonar, sum)

% La funzione si occupa di monitorare la misura dei sonar,
% quando esse sono modificate manda un impulso al blocco di stima relativa

if nnz(isnan(sum)) > 0 || nnz(sum) == 0 
    pulse = 0;
else
    pulse = 1;
end

prev = sonar;

== matlab function controllo_test/Navigation1/Relative estimation/Subsystem/MATLAB Function9 ==
  data: sonar input; orientation input; distance output; alpha output; flag_sonar output; pylonRadius parameter; a parameter; s_data parameter
function [distance, alpha, flag_sonar] = relative_values(sonar, orientation, pylonRadius, a, s_data)

% Chiamando la funzione "fcn_sonar" si occupa di calcolate la distanza
% e l'angolo dell'AUV rispetto al pilone

distance = 0;
alpha = 0;
flag_sonar = 0;

coder.extrinsic('fcn_sonar');

[distance, alpha, flag_sonar] = fcn_sonar(sonar, orientation, pylonRadius, a, s_data);
end

== matlab function controllo_test/Navigation1/flag_function ==
  data: flag_depth input; flag_AHRS input; error_flag output; flag_DVL input; flag_sonar input
function error_flag = fcn(flag_depth, flag_AHRS, flag_DVL, flag_sonar)

% Funzione che rileva la presenza di errore in un sensore

flag_ahrs = flag_AHRS(1) & flag_AHRS(2) & flag_AHRS(3);
error_flag = ~(flag_depth & flag_ahrs & flag_DVL & flag_sonar); % Vale 1 se vi è un errore

== matlab function controllo_test/Navigation1/z_EKF/EXTENDED KALMAN FILTER/Correzione  ==
  data: prev_pos output; prev_pos input; P input; hat input; meas_pos input; GPS_flag input; meas_depth input; P output; hat output; R parameter; H parameter
function [prev_pos, P, hat] = EKF_pos(prev_pos, P, hat, meas_pos, GPS_flag, meas_depth, R, H)
%% EKF: Correction

% Il filtro corregge i valori di posizione x e y solo quando è disponibile una nuova misura del GPS
if nnz(round(10.^4*(meas_pos - prev_pos))/10.^4) ~= 0 && GPS_flag == 1       % Se il flag è 0 il GPS non funziona

    z_tilde = [ meas_pos(1) - hat(1);
                meas_pos(2) - hat(2);
                meas_depth - hat(3)];

else
        z_tilde = [ 0;
                    0;
                meas_depth - hat(3)];
end
            
    S = H * P * H' + R;

    K = P * H' * S^(-1);
    
    hat = hat + K * z_tilde;
    P = (eye(3) - K * H) * P;  

prev_pos = meas_pos;

== matlab function controllo_test/Navigation1/z_EKF/EXTENDED KALMAN FILTER/Predizione ==
  data: P input; hat input; dT input; P output; hat output; orientation input; dvl input; ahrs_flag input; init input; P0 input; Q parameter
function [P, hat]  = EKF_pos(P, hat, dT, orientation, dvl, ahrs_flag, init, P0, Q)

dvl_flag = dvl(4);

%% Inizializzazione stato e matrice P
if nnz(hat) == 0           
    hat= init;
    P = P0;
end

if (ahrs_flag && dvl_flag) == 1
    %% Calcolo variabili e matrici
    phi     =   orientation(1);             % roll
    theta   =   orientation(2);             % pitch
    psi_    =   orientation(3);             % yaw
    vel     =   [dvl(1); dvl(2); dvl(3)];  
    
    J       =   zeros(3,3);
    Lk      =   zeros(3,6);
    
    J = [ cos(psi_)*cos(theta), cos(psi_)*sin(phi)*sin(theta) - cos(phi)*sin(psi_), sin(phi)*sin(psi_) + cos(phi)*cos(psi_)*sin(theta);
       cos(theta)*sin(psi_), cos(phi)*cos(psi_) + sin(phi)*sin(psi_)*sin(theta), cos(phi)*sin(psi_)*sin(theta) - cos(psi_)*sin(phi);
         -sin(theta),                                cos(theta)*sin(phi),                                cos(phi)*cos(theta)];
     
    x = dvl(1);
    y = dvl(2);
    z = dvl(3);
    n_ahrs1 = 0;
    n_ahrs2 = 0;
    n_ahrs3 = 0;

    % Matrice Lk: derivata della funzione f rispetto al rumore di AHRS e
    % DVL
    Lk = [  dT*(y*(sin(n_ahrs1 + phi)*sin(n_ahrs3 + psi_) + cos(n_ahrs1 + phi)*cos(n_ahrs3 + psi_)*sin(n_ahrs2 + theta)) + z*(cos(n_ahrs1 + phi)*sin(n_ahrs3 + psi_) - cos(n_ahrs3 + psi_)*sin(n_ahrs1 + phi)*sin(n_ahrs2 + theta))), dT*(z*cos(n_ahrs1 + phi)*cos(n_ahrs3 + psi_)*cos(n_ahrs2 + theta) - x*cos(n_ahrs3 + psi_)*sin(n_ahrs2 + theta) + y*cos(n_ahrs3 + psi_)*cos(n_ahrs2 + theta)*sin(n_ahrs1 + phi)), -dT*(y*(cos(n_ahrs1 + phi)*cos(n_ahrs3 + psi_) + sin(n_ahrs1 + phi)*sin(n_ahrs3 + psi_)*sin(n_ahrs2 + theta)) - z*(cos(n_ahrs3 + psi_)*sin(n_ahrs1 + phi) - cos(n_ahrs1 + phi)*sin(n_ahrs3 + psi_)*sin(n_ahrs2 + theta)) + x*cos(n_ahrs2 + theta)*sin(n_ahrs3 + psi_)), dT*cos(n_ahrs3 + psi_)*cos(n_ahrs2 + theta), -dT*(cos(n_ahrs1 + phi)*sin(n_ahrs3 + psi_) - cos(n_ahrs3 + psi_)*sin(n_ahrs1 + phi)*sin(n_ahrs2 + theta)),  dT*(sin(n_ahrs1 + phi)*sin(n_ahrs3 + psi_) + cos(n_ahrs1 + phi)*cos(n_ahrs3 + psi_)*sin(n_ahrs2 + theta));
     -dT*(y*(cos(n_ahrs3 + psi_)*sin(n_ahrs1 + phi) - cos(n_ahrs1 + phi)*sin(n_ahrs3 + psi_)*sin(n_ahrs2 + theta)) + z*(cos(n_ahrs1 + phi)*cos(n_ahrs3 + psi_) + sin(n_ahrs1 + phi)*sin(n_ahrs3 + psi_)*sin(n_ahrs2 + theta))), dT*(z*cos(n_ahrs1 + phi)*cos(n_ahrs2 + theta)*sin(n_ahrs3 + psi_) - x*sin(n_ahrs3 + psi_)*sin(n_ahrs2 + theta) + y*cos(n_ahrs2 + theta)*sin(n_ahrs1 + phi)*sin(n_ahrs3 + psi_)),  dT*(z*(sin(n_ahrs1 + phi)*sin(n_ahrs3 + psi_) + cos(n_ahrs1 + phi)*cos(n_ahrs3 + psi_)*sin(n_ahrs2 + theta)) - y*(cos(n_ahrs1 + phi)*sin(n_ahrs3 + psi_) - cos(n_ahrs3 + psi_)*sin(n_ahrs1 + phi)*sin(n_ahrs2 + theta)) + x*cos(n_ahrs3 + psi_)*cos(n_ahrs2 + theta)), dT*cos(n_ahrs2 + theta)*sin(n_ahrs3 + psi_),  dT*(cos(n_ahrs1 + phi)*cos(n_ahrs3 + psi_) + sin(n_ahrs1 + phi)*sin(n_ahrs3 + psi_)*sin(n_ahrs2 + theta)), -dT*(cos(n_ahrs3 + psi_)*sin(n_ahrs1 + phi) - cos(n_ahrs1 + phi)*sin(n_ahrs3 + psi_)*sin(n_ahrs2 + theta));
                                                                                                                                    dT*(y*cos(n_ahrs1 + phi)*cos(n_ahrs2 + theta) - z*cos(n_ahrs2 + theta)*sin(n_ahrs1 + phi)),                                                            -dT*(x*cos(n_ahrs2 + theta) + z*cos(n_ahrs1 + phi)*sin(n_ahrs2 + theta) + y*sin(n_ahrs1 + phi)*sin(n_ahrs2 + theta)),                                                                                                                                                                                                                                                                      0,                    -dT*sin(n_ahrs2 + theta),                                                                 dT*cos(n_ahrs2 + theta)*sin(n_ahrs1 + phi),                                                                 dT*cos(n_ahrs1 + phi)*cos(n_ahrs2 + theta)];

    %% EKF: Predizione

    hat  =  hat + dT * J * vel;        
    P =  P + Lk * Q * Lk';            

 
end

== matlab function controllo_test/Navigation1/z_EKF/Trigger & Init/Depth trigger/MATLAB Function ==
  data: count input; count output; dT output; depth input; sum input; pulse output; prev output
function [count, dT, pulse, prev] = fcn(count, depth, sum)

% La funzione si occupa di monitorare la misura del profondimetro,
% quando essa è modificata manda un impulso al blocco EKF e il tempo
% trascorso dalla precedente variazione

dT = 0;  

if nnz(round(10.^4*sum )/10.^4) == 0
    pulse = 0;
    count = count + 1;
else
    pulse = 1;
    dT = count * (1/200);
    count = 1;
end

prev = depth;

== matlab function controllo_test/Navigation1/Geodetic to NED1/MATLAB Function2 ==
  data: GPS_geodetic input; GPS_flag input; GPS_NED output; depth input; pylonCenter parameter
function GPS_NED = Geo2NED(GPS_geodetic, GPS_flag, depth, pylonCenter)

% Funzione che trasforma le coordinate dal sistema di riferimento geodetico
% ad un sistema NED con origine in corrispondenza del centro del pilone.

%% GPS non funzionante
if GPS_flag == 0            
    GPS_NED = [0;0;0];
    return
end

%% Variabili
phi = GPS_geodetic(1);                  % Coordinate geodetiche in radianti                     
lambda = GPS_geodetic(2);  
h = -depth;

phi_pyl = pylonCenter(1) * pi/180;      % Origine del sistema NED in coordinate geodetiche
lambda_pyl = pylonCenter(2) * pi/180;

%% Trasformazione coordinate
coder.extrinsic('wgs84Ellipsoid');
coder.extrinsic('geodetic2ned');
    
[x_gps2, y_gps2, z_gps2] = geodetic2ned(phi, lambda, -depth, phi_pyl, lambda_pyl, 0, wgs84Ellipsoid, 'radians');
eta_NED_GPS = [x_gps2; y_gps2];

GPS_NED = zeros(3,1);
GPS_NED(1) = eta_NED_GPS(1);            % Coordiante NED in radianti
GPS_NED(2) = eta_NED_GPS(2);
GPS_NED(3) = GPS_flag;

== matlab function controllo_test/Env. & Sensor Model/GPS SENSOR/NED2Geodetic ==
  data: depth input; u input; data_GDT output; enableGps input; pylonCenter parameter
function data_GDT= fcn(depth, u, enableGps, pylonCenter)

lat_origin = pylonCenter(1);
lon_origin= pylonCenter(2);
h_origin = pylonCenter(3);

xNorth = u(1);
yEast = u(2);

if enableGps==1
    [lat,lon, h] = ned2geodeticS(xNorth, yEast, depth, lat_origin, lon_origin, h_origin);
else
    lat=NaN;
    lon=NaN;
end

data_GDT = [lat, lon];

== matlab function controllo_test/Env. & Sensor Model/GPS SENSOR/Threshold ==
  data: depth output; x_out output; x_in input; y_out output; y_in input; h_in input; flag_enable_gps output; gpsThreshold parameter
function [depth, x_out, y_out, flag_enable_gps] = fcn(x_in, y_in, h_in, gpsThreshold)


if (h_in > gpsThreshold) % gps does not work
    flag_enable_gps=0;
    x_in = NaN;
    y_in = NaN;
else % ok gps work 
    flag_enable_gps=1;
end

x_out=x_in;
y_out=y_in;
depth=h_in;

== matlab function controllo_test/Navigation1/z_EKF/Trigger & Init/Initialization/MATLAB Function1 ==
  data: init_counter output; init_counter input; depth input; gps input; GPS_flag input; pulse output; init output; P0 output; prev output; diff_ input; store_gps input; gps_store output; store_depth input; depth_store output; num_cycle parameter
function [init_counter, pulse, init, P0, prev, gps_store, depth_store] = fcn_init(init_counter, depth, gps, GPS_flag, diff_, store_gps, store_depth, num_cycle)

% La funzione si occupa di valutare i valori iniziali dello stato e della varianza dell'errore di stima

%% Variabili
pulse = 0;
gps_store = store_gps;
depth_store = store_depth;
init = zeros(3,1);
P0 = zeros(3);
coder.extrinsic('init_position');

%%
if nnz(round(10.^4*diff_)/10.^4) ~= 0 && init_counter < num_cycle && GPS_flag == 1
    
    init_counter = init_counter + 1;
    gps_store(1, init_counter) = gps(1);
    gps_store(2, init_counter) = gps(2);
    pulse = 0;
    depth_store(init_counter) = depth;

        
elseif init_counter < num_cycle

    init_counter = init_counter;
    pulse = 0;
    
    
elseif init_counter >= num_cycle && init_counter < 300
   
    [init, P0] = init_position(store_gps, store_depth, num_cycle); 
    pulse = 1;
    init_counter = init_counter + 1;

else 
    
    pulse = 1;
   
end

prev = gps;

== matlab function controllo_test/Env. & Sensor Model/AHRS SENSOR/    ==
  data: ni_1 input; ni_1_dot input; lin_acc output; ang_vel output; m output; ni_2 input; eta_2 input; eta_2_dot input
function [lin_acc, ang_vel, m] = IMU(ni_1, ni_1_dot, ni_2, eta_2, eta_2_dot)

% questa funzione, partendo dalle informazioni cinematiche dell' AUV
% restituisce in output delle misure di accelerazione, velocità angolare
% e campo magnetico locale


% definisco R^T
% R = Rz(psi)*Ry(theta)*Rx(phi);

% yaw = psi; pitch = theta; roll = phi;

phi = eta_2(1);
theta = eta_2(2);
psi = eta_2(3);

R = [cos(psi)*cos(theta) cos(psi)*sin(theta)*sin(phi)-sin(psi)*cos(phi) cos(psi)*sin(theta)*cos(phi)+sin(psi)*sin(phi);
     sin(psi)*cos(theta) sin(psi)*sin(theta)*sin(phi)+cos(psi)*cos(phi) sin(psi)*sin(theta)*cos(phi)-cos(psi)*sin(phi);
    -sin(theta) cos(theta)*sin(phi) cos(theta)*cos(phi)];

% Rx_phi = [1 0 0; 0 cos(phi) sin(phi); 0 -sin(phi) cos(phi)];
% Ry_theta = [cos(theta) 0 -sin(theta); 0 1 0; sin(theta) 0 cos(theta)];
% Rz_psi = [cos(psi) sin(psi) 0; -sin(psi) cos(psi) 0; 0 0 1];

% R = Rz_psi'*Ry_theta'*Rx_phi;

% Definisco la matrice Jacobiana
 
%J_2 = [1 sin(phi)*tan(theta) cos(phi)*tan(theta);
%       0 cos(phi) -sin(phi);
%       0 sin(phi)/cos(theta) cos(phi)/cos(theta)];
  
% accelerometro

g = [0 0 9.82]; % [m/s^2]
 
%lin_acc = J_1' * (eta_1_ddot - g);  
 
% eta_1_ddot = J_1 * ni_1_dot + J_1_dot * ni_1

dphi = eta_2_dot(1);
dtheta = eta_2_dot(2);
dpsi = eta_2_dot(3);


J_1_dot = [-dtheta*(sin(theta)*cos(psi)) - dpsi*(sin(psi)*cos(theta)), ...
           dphi*(sin(psi)*sin(phi) + cos(psi)*sin(theta)*cos(phi)) + dtheta*(cos(psi)*cos(theta)*sin(phi)) - dpsi*(cos(psi)*cos(phi) + sin(psi)*sin(theta)*sin(phi)), ... 
           dphi*(sin(psi)*cos(phi) - cos(psi)*sin(theta)*sin(phi)) + dtheta*(cos(psi)*cos(theta)*cos(phi)) + dpsi*(cos(psi)*sin(phi) - sin(psi)*sin(theta)*cos(phi)); ...
          -dtheta*(sin(theta)*sin(psi)) + dpsi*(cos(psi)*cos(theta)), ...
           dphi*(-cos(psi)*sin(phi) + sin(psi)*sin(theta)*cos(phi)) + dtheta*(sin(psi)*cos(theta)*sin(phi)) + dpsi*(-sin(psi)*cos(phi) + cos(psi)*sin(theta)*sin(phi)), ... 
          -dphi*(cos(psi)*cos(phi) + sin(psi)*sin(theta)*sin(phi)) + dtheta*(sin(psi)*cos(theta)*cos(phi)) + dpsi*(sin(psi)*sin(phi) + cos(psi)*sin(theta)*cos(phi)); ...
          -dtheta*(cos(theta)), ...
           dphi*(cos(theta)*cos(phi)) - dtheta*(sin(theta)*sin(phi)), ...
          -dphi*(cos(theta)*sin(phi)) - dtheta*(sin(theta)*cos(phi))];

% J_1 = R;      

eta_1_ddot = R * ni_1_dot + J_1_dot * ni_1;

lin_acc = R' * (eta_1_ddot - g');
 
 
 %  giroscopio
 
 % se mi fosse stata fornita la eta_2_dot (espressa in terna NED, globale) la
 % misura del giroscopio sarebbe stata:
 
 %ang_vel = inv(J_2) * eta_2_dot;
 
 %avendo a disposizione in ingresso l'accelerazione in terna Body, la
 %misura della velocità angolare sarà:
 
 ang_vel = ni_2;
 
 % magnetometro ( campo magnetico terrestre espresso in terna NED)
 
 
% gaussian =  normrnd([0 0 0], [0.00131, 0.00094, 0.00157]);
% gaussian = incertezza dell'intensità del campo magnetico 
% calcolata su: https://www.ngdc.noaa.gov/geomag/calculators/magcalc.shtml#igrfwmm

 m_e = [0.238836 -0.010851 0.392423]'; % + gaussian';
 
 m = R' * m_e;
 
end
